simulink model "cartepole"  (R2022a)
settings: Solver=VariableStepAuto  StartTime=0.0  StopTime=30  RelTol=1e-3
libraries: fuzblock x12
settings Model: Creator=Mojtaba  LastModifiedBy=sanam

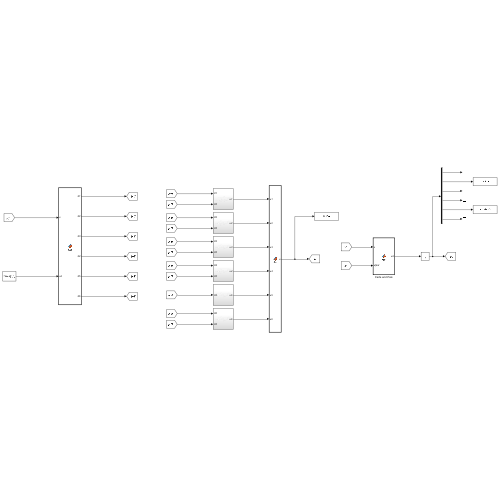
[thumbnail: Simulink's stored preview of the top-level diagram]
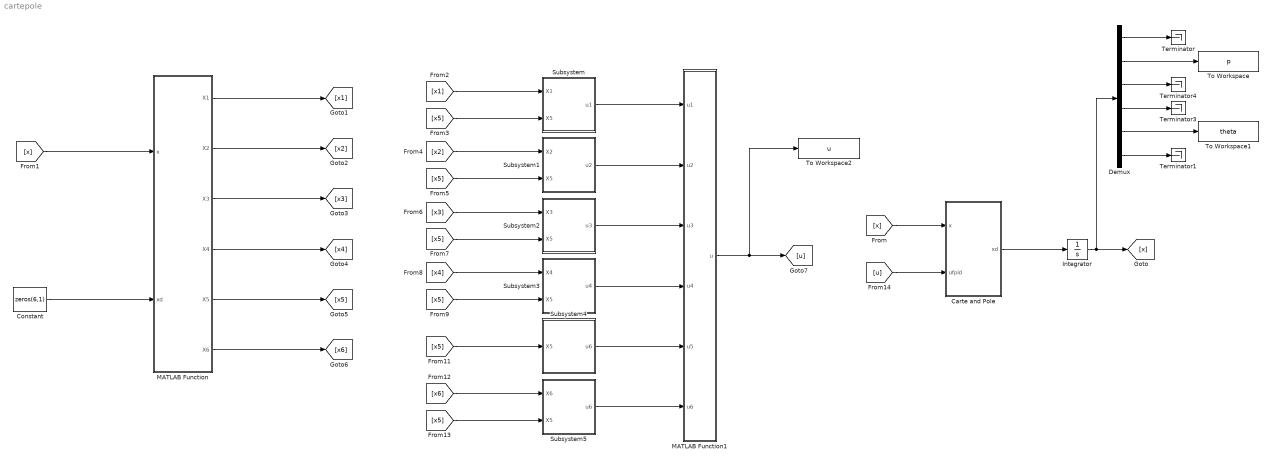
== system cartepole ==
  Carte and Pole : MATLAB Function  TreatAsAtomicUnit=on
  Constant : Constant  Value=zeros(6,1)
  Demux : Demux  Outputs=6
  Integrator : Integrator  InitialCondition=[0;2;0;0;0;0]
  MATLAB Function : MATLAB Function  TreatAsAtomicUnit=on
  MATLAB Function1 : MATLAB Function  TreatAsAtomicUnit=on
  Subsystem : Subsystem
  Subsystem1 : Subsystem
  Subsystem2 : Subsystem
  Subsystem3 : Subsystem
  Subsystem4 : Subsystem
  Subsystem5 : Subsystem
  Terminator{,1,3..4} (4 alike) : Terminator
  To Workspace : ToWorkspace  VariableName=p  SaveFormat=Timeseries  SampleTime=-1
  To Workspace1 : ToWorkspace  VariableName=theta  SaveFormat=Timeseries  SampleTime=-1
  To Workspace2 : ToWorkspace  VariableName=u  SaveFormat=Timeseries  SampleTime=-1
  wires:
  Integrator/1 -> Demux/1, [x]
  [x] -> Carte and Pole/1(x)
  Constant/1 -> MATLAB Function/2(xd)
  [x1] -> Subsystem/1(X1)
  [x5] -> Subsystem/2(X5)
  Subsystem/1(u1) -> MATLAB Function1/1(u1)
  [x5] -> Subsystem1/2(X5)
  [x2] -> Subsystem1/1(X2)
  Subsystem1/1(u2) -> MATLAB Function1/2(u2)
  [x5] -> Subsystem2/2(X5)
  [x3] -> Subsystem2/1(X3)
  Subsystem2/1(u3) -> MATLAB Function1/3(u3)
  [x5] -> Subsystem3/2(X5)
  [x4] -> Subsystem3/1(X4)
  Subsystem3/1(u4) -> MATLAB Function1/4(u4)
  [x5] -> Subsystem4/1(X5)
  Subsystem4/1(u6) -> MATLAB Function1/5(u5)
  [x5] -> Subsystem5/2(X5)
  [x6] -> Subsystem5/1(X6)
  MATLAB Function1/1(u) -> To Workspace2/1, [u]
  [u] -> Carte and Pole/2(ufpid)
  Subsystem5/1(u6) -> MATLAB Function1/6(u6)
  Carte and Pole/1(xd) -> Integrator/1
  MATLAB Function/1(X1) -> [x1]
  MATLAB Function/2(X2) -> [x2]
  MATLAB Function/3(X3) -> [x3]
  MATLAB Function/4(X4) -> [x4]
  MATLAB Function/5(X5) -> [x5]
  MATLAB Function/6(X6) -> [x6]
  [x] -> MATLAB Function/1(x)
  Demux/1 -> Terminator/1
  Demux/3 -> Terminator4/1
  Demux/4 -> Terminator3/1
  Demux/6 -> Terminator1/1
  Demux/2 -> To Workspace/1
  Demux/5 -> To Workspace1/1

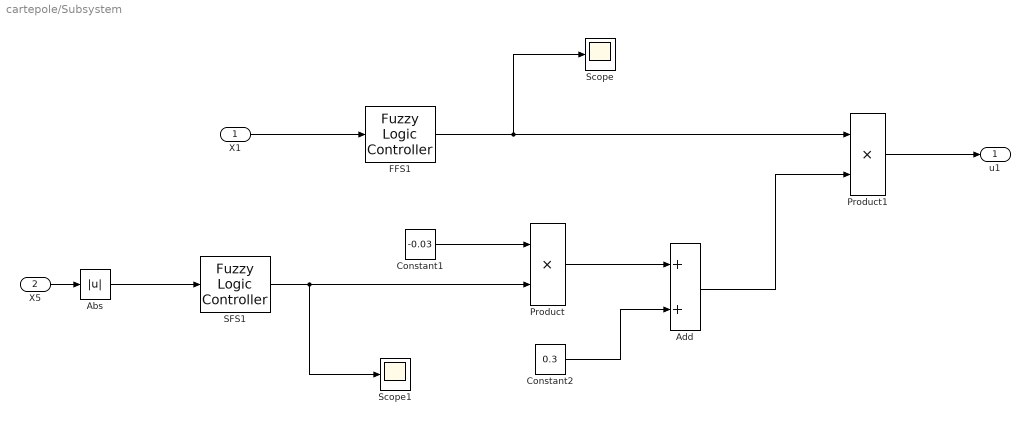
== system cartepole/Subsystem ==
  X1 : Inport
  X5 : Inport  Port=2
  Abs : Abs  SaturateOnIntegerOverflow=off
  Add : Sum
  Constant1 : Constant  Value=-0.03
  Constant2 : Constant  Value=0.3
  FFS1 : fuzblock/Fuzzy Logic  Controller  FIS='FFS1.fis'  OutputSampleNumber=101  DataType=double  FuzzifiedInputs=off  RuleFiringStrengths=off  RuleOutputs=off  AggregatedOutputs=off  SimulateUsing=Interpreted execution  OutOfRangeInputValueMessage=warning  NoRuleFiredMessage=warning  EmptyOutputFuzzySetMessage=warning
  Product : Product
  Product1 : Product
  SFS1 : fuzblock/Fuzzy Logic  Controller  FIS='SFS1.fis'  OutputSampleNumber=101  DataType=double  FuzzifiedInputs=off  RuleFiringStrengths=off  RuleOutputs=off  AggregatedOutputs=off  SimulateUsing=Interpreted execution  OutOfRangeInputValueMessage=warning  NoRuleFiredMessage=warning  EmptyOutputFuzzySetMessage=warning
  Scope : Scope
  Scope1 : Scope
  u1 : Outport
  wires:
  FFS1/1 -> Scope/1, Product1/1
  Product/1 -> Add/1
  SFS1/1 -> Scope1/1, Product/2
  X5/1 -> Abs/1
  Constant1/1 -> Product/1
  Constant2/1 -> Add/2
  Add/1 -> Product1/2
  Product1/1 -> u1/1
  X1/1 -> FFS1/1
  Abs/1 -> SFS1/1

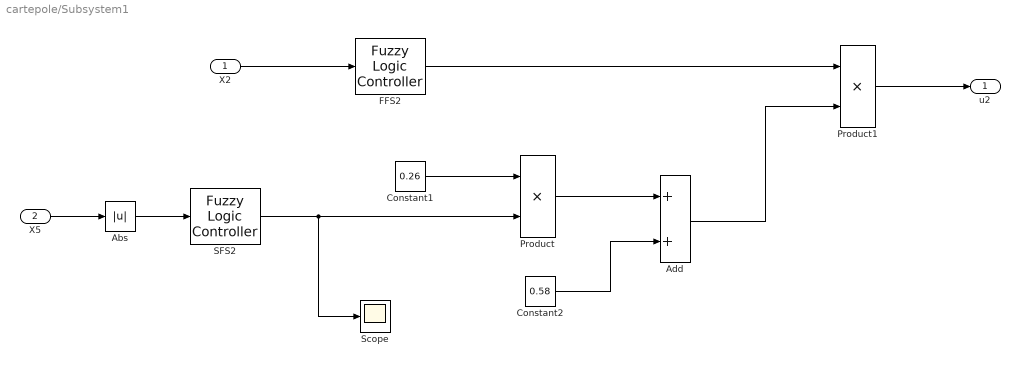
== system cartepole/Subsystem1 ==
  X2 : Inport
  X5 : Inport  Port=2
  Abs : Abs  SaturateOnIntegerOverflow=off
  Add : Sum
  Constant1 : Constant  Value=0.26
  Constant2 : Constant  Value=0.58
  FFS2 : fuzblock/Fuzzy Logic  Controller  FIS='FFS2.fis'  OutputSampleNumber=101  DataType=double  FuzzifiedInputs=off  RuleFiringStrengths=off  RuleOutputs=off  AggregatedOutputs=off  SimulateUsing=Interpreted execution  OutOfRangeInputValueMessage=warning  NoRuleFiredMessage=warning  EmptyOutputFuzzySetMessage=warning
  Product : Product
  Product1 : Product
  SFS2 : fuzblock/Fuzzy Logic  Controller  FIS='SFS2.fis'  OutputSampleNumber=101  DataType=double  FuzzifiedInputs=off  RuleFiringStrengths=off  RuleOutputs=off  AggregatedOutputs=off  SimulateUsing=Interpreted execution  OutOfRangeInputValueMessage=warning  NoRuleFiredMessage=warning  EmptyOutputFuzzySetMessage=warning
  Scope : Scope
  u2 : Outport
  wires:
  FFS2/1 -> Product1/1
  Product/1 -> Add/1
  SFS2/1 -> Scope/1, Product/2
  X5/1 -> Abs/1
  Constant1/1 -> Product/1
  Constant2/1 -> Add/2
  Add/1 -> Product1/2
  X2/1 -> FFS2/1
  Product1/1 -> u2/1
  Abs/1 -> SFS2/1

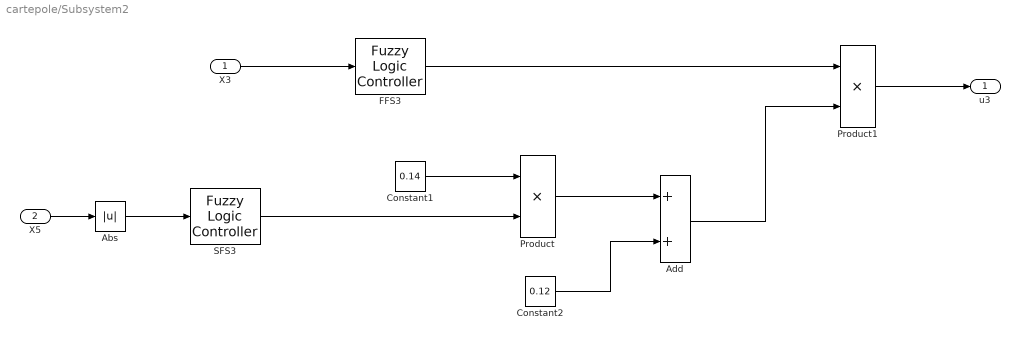
== system cartepole/Subsystem2 ==
  X3 : Inport
  X5 : Inport  Port=2
  Abs : Abs  SaturateOnIntegerOverflow=off
  Add : Sum
  Constant1 : Constant  Value=0.14
  Constant2 : Constant  Value=0.12
  FFS3 : fuzblock/Fuzzy Logic  Controller  FIS='FFS3.fis'  OutputSampleNumber=101  DataType=double  FuzzifiedInputs=off  RuleFiringStrengths=off  RuleOutputs=off  AggregatedOutputs=off  SimulateUsing=Interpreted execution  OutOfRangeInputValueMessage=warning  NoRuleFiredMessage=warning  EmptyOutputFuzzySetMessage=warning
  Product : Product
  Product1 : Product
  SFS3 : fuzblock/Fuzzy Logic  Controller  FIS='SFS3.fis'  OutputSampleNumber=101  DataType=double  FuzzifiedInputs=off  RuleFiringStrengths=off  RuleOutputs=off  AggregatedOutputs=off  SimulateUsing=Interpreted execution  OutOfRangeInputValueMessage=warning  NoRuleFiredMessage=warning  EmptyOutputFuzzySetMessage=warning
  u3 : Outport
  wires:
  FFS3/1 -> Product1/1
  Product/1 -> Add/1
  SFS3/1 -> Product/2
  X5/1 -> Abs/1
  Constant1/1 -> Product/1
  Constant2/1 -> Add/2
  Add/1 -> Product1/2
  X3/1 -> FFS3/1
  Product1/1 -> u3/1
  Abs/1 -> SFS3/1

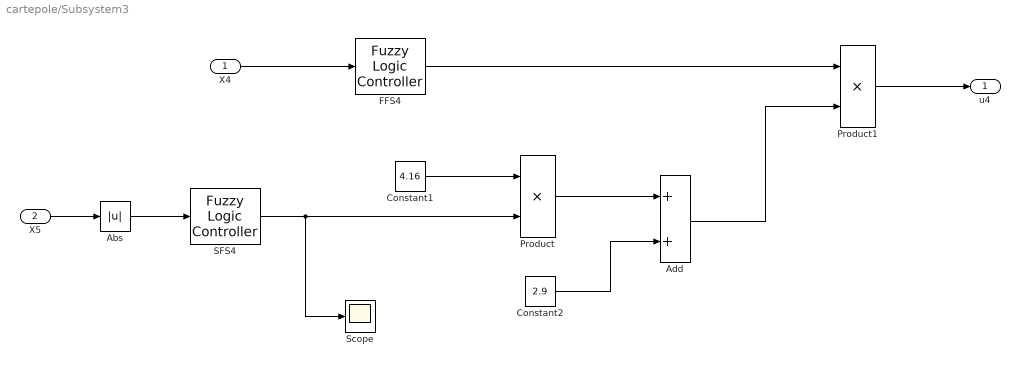
== system cartepole/Subsystem3 ==
  X4 : Inport
  X5 : Inport  Port=2
  Abs : Abs  SaturateOnIntegerOverflow=off
  Add : Sum
  Constant1 : Constant  Value=4.16
  Constant2 : Constant  Value=2.9
  FFS4 : fuzblock/Fuzzy Logic  Controller  FIS='FFS4.fis'  OutputSampleNumber=101  DataType=double  FuzzifiedInputs=off  RuleFiringStrengths=off  RuleOutputs=off  AggregatedOutputs=off  SimulateUsing=Interpreted execution  OutOfRangeInputValueMessage=warning  NoRuleFiredMessage=warning  EmptyOutputFuzzySetMessage=warning
  Product : Product
  Product1 : Product
  SFS4 : fuzblock/Fuzzy Logic  Controller  FIS='SFS4.fis'  OutputSampleNumber=101  DataType=double  FuzzifiedInputs=off  RuleFiringStrengths=off  RuleOutputs=off  AggregatedOutputs=off  SimulateUsing=Interpreted execution  OutOfRangeInputValueMessage=warning  NoRuleFiredMessage=warning  EmptyOutputFuzzySetMessage=warning
  Scope : Scope
  u4 : Outport
  wires:
  FFS4/1 -> Product1/1
  Product/1 -> Add/1
  SFS4/1 -> Scope/1, Product/2
  X5/1 -> Abs/1
  Constant1/1 -> Product/1
  Constant2/1 -> Add/2
  Add/1 -> Product1/2
  X4/1 -> FFS4/1
  Product1/1 -> u4/1
  Abs/1 -> SFS4/1

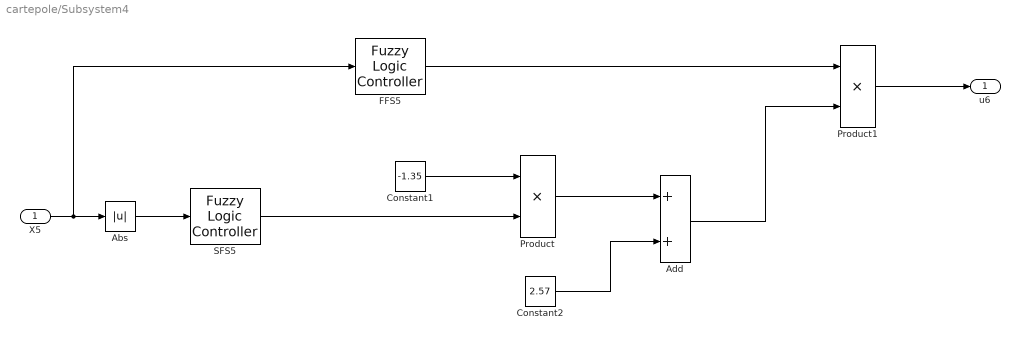
== system cartepole/Subsystem4 ==
  X5 : Inport
  Abs : Abs  SaturateOnIntegerOverflow=off
  Add : Sum
  Constant1 : Constant  Value=-1.35
  Constant2 : Constant  Value=2.57
  FFS5 : fuzblock/Fuzzy Logic  Controller  FIS='FFS5.fis'  OutputSampleNumber=101  DataType=double  FuzzifiedInputs=off  RuleFiringStrengths=off  RuleOutputs=off  AggregatedOutputs=off  SimulateUsing=Interpreted execution  OutOfRangeInputValueMessage=warning  NoRuleFiredMessage=warning  EmptyOutputFuzzySetMessage=warning
  Product : Product
  Product1 : Product
  SFS5 : fuzblock/Fuzzy Logic  Controller  FIS='SFS5.fis'  OutputSampleNumber=101  DataType=double  FuzzifiedInputs=off  RuleFiringStrengths=off  RuleOutputs=off  AggregatedOutputs=off  SimulateUsing=Interpreted execution  OutOfRangeInputValueMessage=warning  NoRuleFiredMessage=warning  EmptyOutputFuzzySetMessage=warning
  u6 : Outport
  wires:
  FFS5/1 -> Product1/1
  Product/1 -> Add/1
  SFS5/1 -> Product/2
  X5/1 -> Abs/1, FFS5/1
  Constant1/1 -> Product/1
  Constant2/1 -> Add/2
  Add/1 -> Product1/2
  Product1/1 -> u6/1
  Abs/1 -> SFS5/1

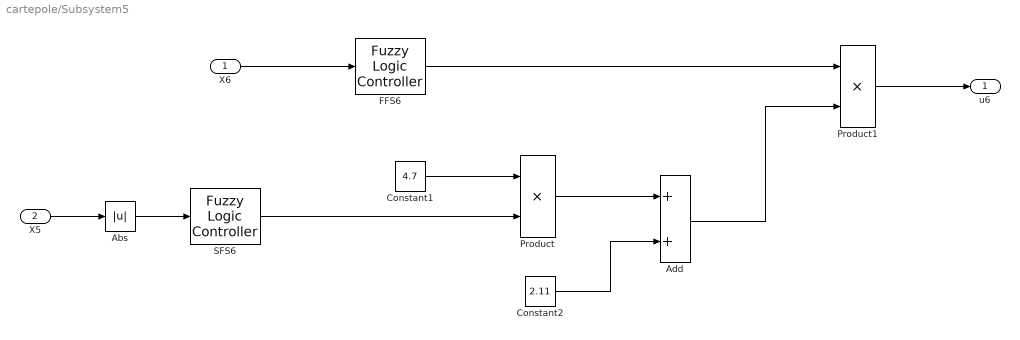
== system cartepole/Subsystem5 ==
  X6 : Inport
  X5 : Inport  Port=2
  Abs : Abs  SaturateOnIntegerOverflow=off
  Add : Sum
  Constant1 : Constant  Value=4.7
  Constant2 : Constant  Value=2.11
  FFS6 : fuzblock/Fuzzy Logic  Controller  FIS='FFS6.fis'  OutputSampleNumber=101  DataType=double  FuzzifiedInputs=off  RuleFiringStrengths=off  RuleOutputs=off  AggregatedOutputs=off  SimulateUsing=Interpreted execution  OutOfRangeInputValueMessage=warning  NoRuleFiredMessage=warning  EmptyOutputFuzzySetMessage=warning
  Product : Product
  Product1 : Product
  SFS6 : fuzblock/Fuzzy Logic  Controller  FIS='SFS6.fis'  OutputSampleNumber=101  DataType=double  FuzzifiedInputs=off  RuleFiringStrengths=off  RuleOutputs=off  AggregatedOutputs=off  SimulateUsing=Interpreted execution  OutOfRangeInputValueMessage=warning  NoRuleFiredMessage=warning  EmptyOutputFuzzySetMessage=warning
  u6 : Outport
  wires:
  FFS6/1 -> Product1/1
  Product/1 -> Add/1
  SFS6/1 -> Product/2
  X5/1 -> Abs/1
  Constant1/1 -> Product/1
  Constant2/1 -> Add/2
  Add/1 -> Product1/2
  X6/1 -> FFS6/1
  Product1/1 -> u6/1
  Abs/1 -> SFS6/1

== matlab function cartepole/MATLAB Function ==
  data: x input; X1 output; xd input; X2 output; X3 output; X4 output; X5 output; X6 output
function [X1,X2,X3,X4,X5,X6] = fcn(x,xd)

e=x-xd;


X1=e(1);

X2=e(2);

X3=e(3);

X4=e(4);

X5=e(5);

X6=e(6);

end

== matlab function cartepole/Carte and Pole ==
  data: x input; ufpid input; xd output
function xd = fcn(x,ufpid)

mc=1;
mp=0.1;
lp=0.5;
g=9.8;

u=11*ufpid;

x1d=x(2);
x2d=x(3);

x3d=( (4/3)*(u+mp*lp*x(6)*x(6)*sin(x(5)) ) - mp*g*sin(x(5))*cos(x(5)) )/ ((4/3)*(mc+mp) - mp*cos(x(5))*cos(x(5)) );

x4d=x(5);
x5d=x(6);

x6d= ( (mc+mp)*g*sin(x(5)) - (u+mp*lp*x(6)*x(6)*sin(x(5)))*cos(x(5)) ) / ( lp*((4/3)*(mc+mp)-mp*cos(x(5))*cos(x(5))) );





xd=[x1d;x2d;x3d;x4d;x5d;x6d];

== matlab function cartepole/MATLAB Function1 ==
  data: u1 input; u output; u2 input; u3 input; u4 input; u5 input; u6 input
function u = fcn(u1,u2,u3,u4,u5,u6)

u= u1 + 0.2*u2 + u3 + u4 + 2*u5 + 0.1*u6;

end
